simulink model "volt_TO_current"  (R2021a)
settings: Solver=VariableStepAuto  StartTime=0.0  StopTime=10.0  RelTol=1e-3
settings Model: Creator=MAC  LastModifiedBy=MAC

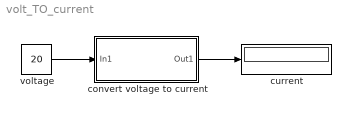
== system volt_TO_current ==
  convert voltage to current : Subsystem
  current : Display
  voltage : Constant  Value=20
  wires:
  voltage/1 -> convert voltage to current/1(In1)
  convert voltage to current/1(Out1) -> current/1

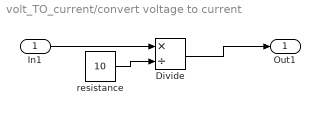
== system volt_TO_current/convert voltage to current ==
  In1 : Inport
  Divide : Product  Inputs=*/
  resistance : Constant  Value=10
  Out1 : Outport
  wires:
  In1/1 -> Divide/1
  resistance/1 -> Divide/2
  Divide/1 -> Out1/1
